simulink model "Simulink_Lab1slx"  (R2022b)
settings: Solver=VariableStepAuto  StartTime=0.0  StopTime=10.0  RelTol=1e-3
settings Model: Creator=ahmed  LastModifiedBy=ahmed

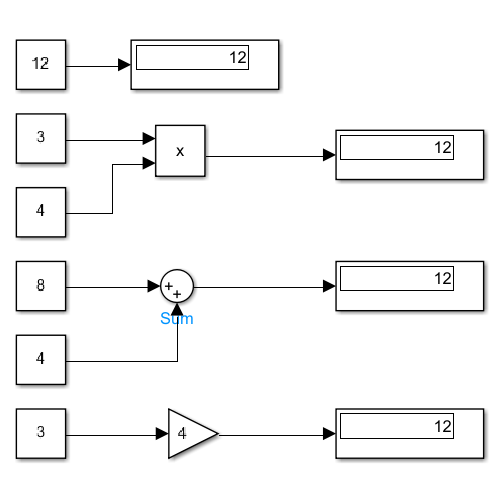
[thumbnail: Simulink's stored preview of the top-level diagram]
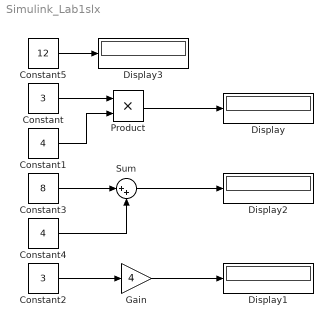
== system Simulink_Lab1slx ==
  Constant : Constant  Value=3
  Constant1 : Constant  Value=4
  Constant2 : Constant  Value=3
  Constant3 : Constant  Value=8
  Constant4 : Constant  Value=4
  Constant5 : Constant  Value=12
  Display{,1..3} (4 alike) : Display
  Gain : Gain  Gain=4
  Product : Product
  Sum : Sum  Inputs=|++
  wires:
  Constant5/1 -> Display3/1
  Product/1 -> Display/1
  Constant4/1 -> Sum/2
  Constant3/1 -> Sum/1
  Constant1/1 -> Product/2
  Constant/1 -> Product/1
  Constant2/1 -> Gain/1
  Sum/1 -> Display2/1
  Gain/1 -> Display1/1
